simulink library "POSH"  (R2016a)
settings: Solver=ode45  StartTime=0.0  StopTime=10.0  RelTol=1e-3
undefined symbols (not defined in the file): BACKWARD, FORWARD, initX, initY, ROB_EAST, ROB_NORTH, ROB_SOUTH, ROB_WEST, ROOM_SIDE_SIZE
settings Model: Creator=oelkawok  LastModifiedBy=omaro
settings DataIOCC: LimitDataPoints=on
settings DebuggingCC: AllowSymbolicDim=off

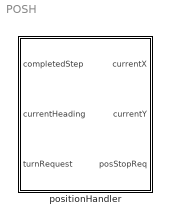
== system POSH ==
  positionHandler : Subsystem

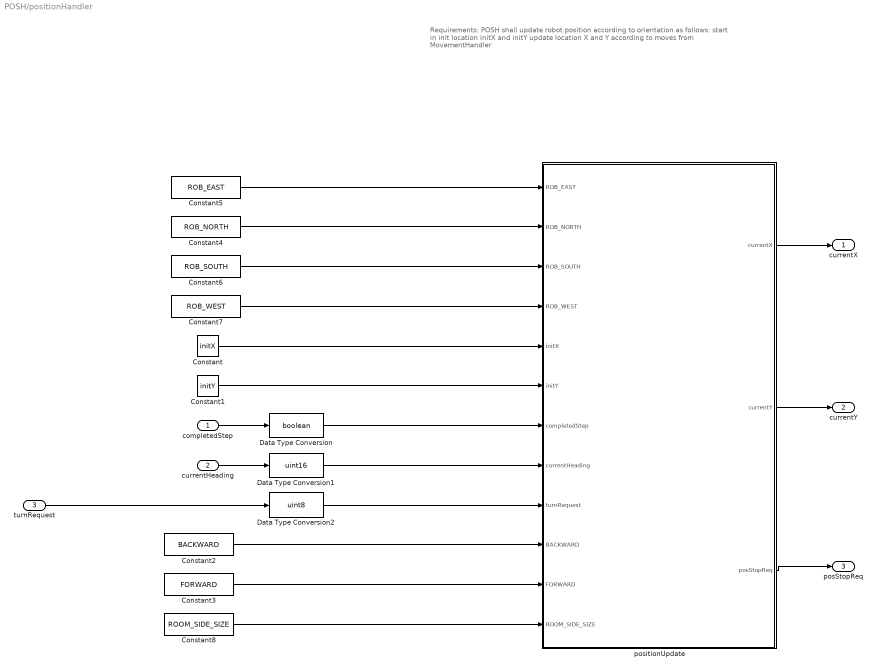
== system POSH/positionHandler ==
  note: Requirements:
      | POSH shall update robot position according to orientation as follows:
      | start in init location initX and initY
      | update location X and Y according to moves from MovementHandler
  completedStep : Inport
  currentHeading : Inport  Port=2
  turnRequest : Inport  Port=3
  Constant : Constant  Value=initX
  Constant1 : Constant  Value=initY
  Constant2 : Constant  Value=BACKWARD
  Constant3 : Constant  Value=FORWARD
  Constant4 : Constant  Value=ROB_NORTH
  Constant5 : Constant  Value=ROB_EAST
  Constant6 : Constant  Value=ROB_SOUTH
  Constant7 : Constant  Value=ROB_WEST
  Constant8 : Constant  Value=ROOM_SIDE_SIZE
  Data Type Conversion : DataTypeConversion  OutDataTypeStr=boolean
  Data Type Conversion1 : DataTypeConversion  OutDataTypeStr=uint16
  Data Type Conversion2 : DataTypeConversion  OutDataTypeStr=uint8
  positionUpdate : Stateflow chart  TreatAsAtomicUnit=on
  currentX : Outport
  currentY : Outport  Port=2
  posStopReq : Outport  Port=3
  wires:
  Constant8/1 -> positionUpdate/12(ROOM_SIDE_SIZE)
  positionUpdate/3(posStopReq) -> posStopReq/1
  Constant2/1 -> positionUpdate/10(BACKWARD)
  Constant3/1 -> positionUpdate/11(FORWARD)
  Data Type Conversion2/1 -> positionUpdate/9(turnRequest)
  Data Type Conversion1/1 -> positionUpdate/8(currentHeading)
  Data Type Conversion/1 -> positionUpdate/7(completedStep)
  turnRequest/1 -> Data Type Conversion2/1
  completedStep/1 -> Data Type Conversion/1
  currentHeading/1 -> Data Type Conversion1/1
  positionUpdate/1(currentX) -> currentX/1
  positionUpdate/2(currentY) -> currentY/1
  Constant5/1 -> positionUpdate/1(ROB_EAST)
  Constant4/1 -> positionUpdate/2(ROB_NORTH)
  Constant7/1 -> positionUpdate/4(ROB_WEST)
  Constant6/1 -> positionUpdate/3(ROB_SOUTH)
  Constant1/1 -> positionUpdate/6(initY)
  Constant/1 -> positionUpdate/5(initX)

== stateflow chart POSH/positionHandler/positionUpdate ==
  state init
    en:
    currentY = initY;
    currentX = initX;
  state inMove
  state North
  state West
  state South
  state East
  (default) -> init
  init -> inMove
  (junction 52) -> inMove
  (junction 15) -> inMove [order 1] : [(((currentY + 1) >=...
      |  ROOM_SIDE_SIZE)...
      | && (turnRequest == BACKWARD))...
      | ||...
      | (((currentY - 1) <= 0)...
      | &&(turnRequest == FORWARD))]
      | /posStopReq = true;
  (junction 24) -> inMove [order 1] : [(((currentX + 1) >=...
      |  ROOM_SIDE_SIZE)...
      | && (turnRequest == BACKWARD))...
      | ||...
      | (((currentX - 1) <= 0)...
      | &&(turnRequest == FORWARD))]
      | /posStopReq = true;
  inMove -> (junction 13) : [(completedStep == true)...
      | && hasChanged(completedStep)]
      | /posStopReq = false;
  (junction 30) -> inMove [order 1] : [(((currentY + 1) >=...
      |  ROOM_SIDE_SIZE)...
      | &&(turnRequest == FORWARD))...
      | ||...
      | (((currentY - 1) <= 0)...
      | && (turnRequest == BACKWARD))]
      | /posStopReq = true;
  (junction 36) -> inMove [order 1] : [(((currentX + 1) >=...
      |  ROOM_SIDE_SIZE)...
      | &&(turnRequest == FORWARD))...
      | ||...
      | (((currentX - 1) <= 0)...
      | && (turnRequest == BACKWARD))]
      | /posStopReq = true;
  (junction 13) -> (junction 36) [order 4] : [currentHeading == ROB_EAST]
  (junction 13) -> (junction 15) [order 1] : [currentHeading == ROB_NORTH]
  (junction 13) -> (junction 30) [order 3] : [currentHeading == ROB_SOUTH]
  (junction 13) -> (junction 24) [order 2] : [currentHeading == ROB_WEST]
  (junction 15) -> North [order 2] : [(turnRequest == FORWARD)]
      | /currentY--;
  (junction 15) -> North [order 3] : [turnRequest == BACKWARD]
      | /currentY++;
  (junction 24) -> West [order 2] : [turnRequest == FORWARD]
      | /currentX--;
  (junction 30) -> South [order 3] : [turnRequest == BACKWARD]
      | /currentY--;
  (junction 30) -> South [order 2] : [turnRequest == FORWARD]
      | /currentY++;
  (junction 36) -> East [order 2] : [turnRequest == FORWARD]
      | /currentX++;
  (junction 24) -> West [order 3] : [turnRequest == BACKWARD]
      | /currentX++;
  (junction 36) -> East [order 3] : [turnRequest == BACKWARD]
      | /currentX--;
  East -> (junction 52)
  North -> (junction 52)
  West -> (junction 52)
  South -> (junction 52)
  data: ROB_EAST input; ROB_NORTH input; ROB_SOUTH input; ROB_WEST input; currentX output int32; currentY output int32; initX input; initY input; completedStep input; currentHeading input; turnRequest input; BACKWARD input; FORWARD input; posStopReq output boolean; ROOM_SIDE_SIZE input
